simulink model "sch_2"  (R2022b)
settings: Solver=FixedStepAuto  StartTime=0.0  StopTime=3*t_final  FixedStep=1  RelTol=1e-3
values from neighbouring files (symbols this model uses):
  a = 7068e3    (= 7068000)    [prgBE_DSAS.m]
  Kp = lqr(Ap,Bp,eye(9),1e11*eye(3))    [prgBE_DSAS.m]
  n = sqrt(mu/a^3)    [prgBE_DSAS.m]
  X_init_chasseur = [x_init(2);y_init(2);z_init(2);Vx_init(2);Vy_init(2);Vz_init(2)]    [initialisation_a_distribuer.m]
  X_init_cible = [x_init(1);y_init(1);z_init(1);Vx_init(1);Vy_init(1);Vz_init(1)]    [initialisation_a_distribuer.m]
undefined symbols (not defined in the file or in its folder): ecc, inc, nu, W, w
settings Model: Creator=franc  LastModifiedBy=Utilisateur
settings DataIOCC: ReturnWorkspaceOutputs=off
settings OptimizationCC: ReuseModelBlockBuffer=on

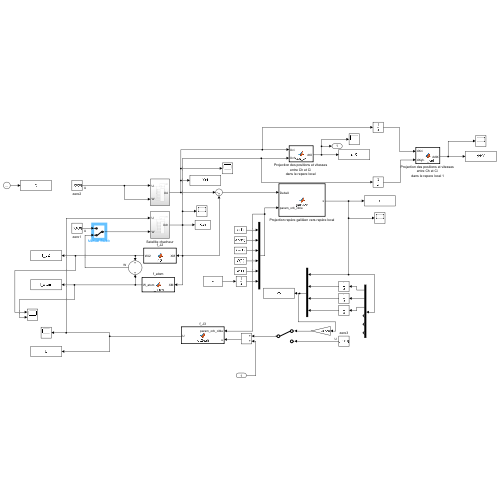
[thumbnail: Simulink's stored preview of the top-level diagram]
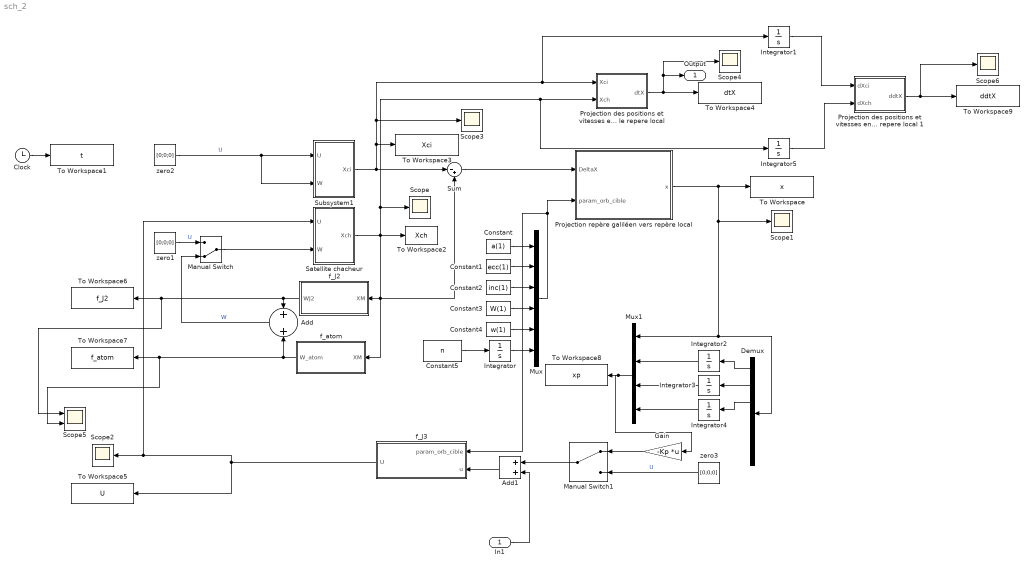
== system sch_2 ==
  In1 : Inport
  Add : Sum
  Add1 : Sum
  Clock : Clock
  Constant : Constant  Value=a(1)
  Constant1 : Constant  Value=ecc(1)
  Constant2 : Constant  Value=inc(1)
  Constant3 : Constant  Value=W(1)
  Constant4 : Constant  Value=w(1)
  Constant5 : Constant  Value=n
  Demux : Demux  Outputs=6
  Gain : Gain  Gain=-Kp  Multiplication=Matrix(K*u)
  Integrator : Integrator  InitialCondition=nu(1)
  Integrator{1..5} (5 alike) : Integrator
  Manual Switch : ManualSwitch  CurrentSetting=0
  Manual Switch1 : ManualSwitch
  Mux : Mux  Inputs=6
  Mux1 : Mux
  "Projection des positions et vitesses entre Ch et Ci dans le repere local " : MATLAB Function  TreatAsAtomicUnit=on
  Projection des positions et vitesses entre Ch et Ci dans le repere local 1 : MATLAB Function  TreatAsAtomicUnit=on
  Projection repère galiléen vers repère local : MATLAB Function  TreatAsAtomicUnit=on
  Satellite chacheur : Subsystem
  Scope{,1..4,6} (6 alike) : Scope
  Scope5 : Scope  NumInputPorts=2
  Subsystem1 : Subsystem
  Sum : Sum  Inputs=|-+
  To Workspace : ToWorkspace  VariableName=x  SampleTime=-1
  To Workspace1 : ToWorkspace  VariableName=t  SampleTime=-1
  To Workspace2 : ToWorkspace  VariableName=Xch  SampleTime=-1
  To Workspace3 : ToWorkspace  VariableName=Xci  SampleTime=-1
  To Workspace4 : ToWorkspace  VariableName=dtX  SampleTime=-1
  To Workspace5 : ToWorkspace  VariableName=U  SampleTime=-1
  To Workspace6 : ToWorkspace  VariableName=f_J2  SampleTime=-1
  To Workspace7 : ToWorkspace  VariableName=f_atom  SampleTime=-1
  To Workspace8 : ToWorkspace  VariableName=xp  SampleTime=-1
  To Workspace9 : ToWorkspace  VariableName=ddtX  SampleTime=-1
  f_J2 : MATLAB Function  TreatAsAtomicUnit=on
  f_J3 : MATLAB Function  TreatAsAtomicUnit=on
  f_atom : MATLAB Function  TreatAsAtomicUnit=on
  zero1 : Constant  Value=[0;0;0]
  zero2 : Constant  Value=[0;0;0]
  zero3 : Constant  Value=[0;0;0]
  Output : Outport
  wires:
  Integrator3/1 -> Mux1/3
  Integrator4/1 -> Mux1/4
  Gain/1 -> Manual Switch1/1
  Demux/3 -> Integrator4/1
  Projection repère galiléen vers repère local/1(x) -> Scope1/1, Demux/1, Mux1/1, To Workspace/1
  Demux/2 -> Integrator3/1
  Demux/1 -> Integrator2/1
  Constant1/1 -> Mux/2
  Constant/1 -> Mux/1
  zero1/1 -> Manual Switch/1  "U"
  zero2/1 -> Subsystem1/2(W), Subsystem1/1(U)  "U"
  Manual Switch/1 -> Satellite chacheur/2(W)
  Integrator/1 -> Mux/6
  Add/1 -> Manual Switch/2  "W"
  zero3/1 -> Manual Switch1/2  "U"
  "Projection des positions et vitesses entre Ch et Ci dans le repere local "/1(dtX) -> Output/1, Scope4/1, To Workspace4/1
  Mux1/1 -> Gain/1, To Workspace8/1
  Constant5/1 -> Integrator/1
  Constant3/1 -> Mux/4
  Clock/1 -> To Workspace1/1
  f_J3/1(U) -> Satellite chacheur/1(U), Scope2/1, To Workspace5/1
  Integrator2/1 -> Mux1/2
  Mux/1 -> f_J3/1(param_orb_cible), Projection repère galiléen vers repère local/2(param_orb_cible)
  f_J2/1(WJ2) -> Scope5/1, To Workspace6/1, Add/1
  Constant4/1 -> Mux/5
  f_atom/1(W_atom) -> Scope5/2, To Workspace7/1, Add/2
  Constant2/1 -> Mux/3
  Sum/1 -> Projection repère galiléen vers repère local/1(DeltaX)
  Integrator5/1 -> Projection des positions et vitesses entre Ch et Ci dans le repere local 1/2(dXch)
  Satellite chacheur/1(Xch) -> Integrator5/1, "Projection des positions et vitesses entre Ch et Ci dans le repere local "/2(Xch), Scope/1, f_atom/1(XM), Sum/2, f_J2/1(XM), To Workspace2/1
  Projection des positions et vitesses entre Ch et Ci dans le repere local 1/1(ddtX) -> Scope6/1, To Workspace9/1
  Subsystem1/1(Xci) -> Scope3/1, Integrator1/1, "Projection des positions et vitesses entre Ch et Ci dans le repere local "/1(Xci), To Workspace3/1, Sum/1
  Integrator1/1 -> Projection des positions et vitesses entre Ch et Ci dans le repere local 1/1(dXci)
  Add1/1 -> f_J3/2(u)
  In1/1 -> Add1/2
  Manual Switch1/1 -> Add1/1

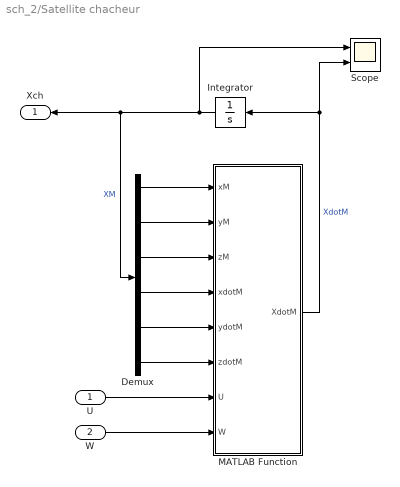
== system sch_2/Satellite chacheur ==
  U : Inport
  W : Inport  Port=2
  Demux : Demux  Outputs=6
  Integrator : Integrator  InitialCondition=X_init_chasseur
  MATLAB Function : MATLAB Function  TreatAsAtomicUnit=on
  Scope : Scope  NumInputPorts=2
  Xch : Outport
  wires:
  Demux/5 -> MATLAB Function/5(ydotM)
  Demux/1 -> MATLAB Function/1(xM)
  Demux/6 -> MATLAB Function/6(zdotM)
  MATLAB Function/1(XdotM) -> Scope/2, Integrator/1  "XdotM"
  Demux/4 -> MATLAB Function/4(xdotM)
  Integrator/1 -> Scope/1, Xch/1, Demux/1  "XM"
  Demux/2 -> MATLAB Function/2(yM)
  Demux/3 -> MATLAB Function/3(zM)
  U/1 -> MATLAB Function/7(U)
  W/1 -> MATLAB Function/8(W)

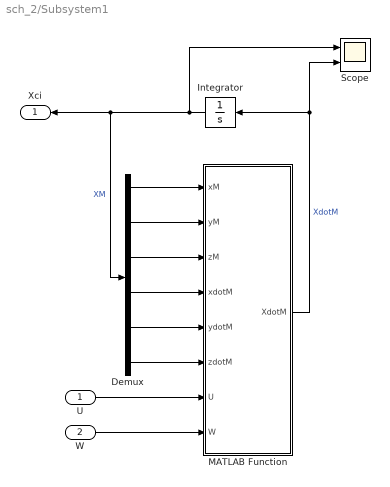
== system sch_2/Subsystem1 ==
  U : Inport
  W : Inport  Port=2
  Demux : Demux  Outputs=6
  Integrator : Integrator  InitialCondition=X_init_cible
  MATLAB Function : MATLAB Function  TreatAsAtomicUnit=on
  Scope : Scope  NumInputPorts=2
  Xci : Outport
  wires:
  Demux/5 -> MATLAB Function/5(ydotM)
  Demux/1 -> MATLAB Function/1(xM)
  Demux/6 -> MATLAB Function/6(zdotM)
  MATLAB Function/1(XdotM) -> Scope/2, Integrator/1  "XdotM"
  Demux/4 -> MATLAB Function/4(xdotM)
  Integrator/1 -> Scope/1, Xci/1, Demux/1  "XM"
  Demux/2 -> MATLAB Function/2(yM)
  Demux/3 -> MATLAB Function/3(zM)
  U/1 -> MATLAB Function/7(U)
  W/1 -> MATLAB Function/8(W)

== matlab function sch_2/Subsystem1/MATLAB Function ==
  data: xM input; yM input; zM input; xdotM input; ydotM input; zdotM input; XdotM output; U input; W input
function XdotM = f(xM,yM,zM,xdotM,ydotM,zdotM, U, W)
mu = 3.986e14; 
BW = [  zeros(3,3);
        eye(3)];

BU = [  eye(3);
        zeros(3,3)];


XdotM = [   xdotM;
            ydotM;
            zdotM;
            -mu/sqrt((xM^2 + yM^2 + zM^2)^3)*xM;
            -mu/sqrt((xM^2 + yM^2 + zM^2)^3)*yM;
            -mu/sqrt((xM^2 + yM^2 + zM^2)^3)*zM] + BU*U + BW*W;

== matlab function sch_2/Satellite chacheur/MATLAB Function ==
  data: xM input; yM input; zM input; xdotM input; ydotM input; zdotM input; XdotM output; U input; W input
function XdotM = f(xM,yM,zM,xdotM,ydotM,zdotM, U, W)
mu = 3.986e14; 
BW = [  zeros(3,3);
        eye(3)];

BU = [  zeros(3,3);  
        eye(3)     ];


XdotM = [   xdotM;
            ydotM;
            zdotM;
            -mu/sqrt((xM^2 + yM^2 + zM^2)^3)*xM;
            -mu/sqrt((xM^2 + yM^2 + zM^2)^3)*yM;
            -mu/sqrt((xM^2 + yM^2 + zM^2)^3)*zM] + BU*U + BW*W;

== matlab function sch_2/f_atom ==
  data: XM input; W_atom output
function W_atom = f_atom(XM)

rho_0 = 6.3e-13; 
rho = rho_0; 
S = 2; 
m = 191.1; 
CD = 2; 

W_atom = [  -rho*S*CD*sqrt(XM(4)^2+XM(5)^2+XM(6)^2)/2/m*XM(4)
            -rho*S*CD*sqrt(XM(4)^2+XM(5)^2+XM(6)^2)/2/m*XM(5)
            -rho*S*CD*sqrt(XM(4)^2+XM(5)^2+XM(6)^2)/2/m*XM(6) ];

== matlab function sch_2/f_J2 ==
  data: XM input; WJ2 output
function WJ2 = fJ2(XM)

mu = 3.986e14;          % constante gravitationnnelle 
J2 = 1.082616e-3;       % second harmonique 
Req = 6378e3;           % rayon terrestre (m)
WJ2 = 1/2*mu*J2*Req*Req*(3/sqrt(XM(1)^2+XM(2)^2+XM(3)^2)^4 - 15*XM(3)/sqrt(XM(1)^2+XM(2)^2+XM(3)^2)^6)*[XM(1);XM(2);XM(3)]/sqrt(XM(1)^2+XM(2)^2+XM(3)^2);

== matlab function sch_2/Projection repère galiléen vers repère local ==
  data: DeltaX input; x output; param_orb_cible input
function x = gali2loc(DeltaX,param_orb_cible)

mu = 3.986e14;

Delta_pos_gali = DeltaX(1:3);
Delta_vit_gali = DeltaX(4:6);
a1 = param_orb_cible(1);
ecc1 = param_orb_cible(2);
inc1 = param_orb_cible(3);
W1 = param_orb_cible(4);
w1 = param_orb_cible(5);
nu1 = param_orb_cible(6);

 P_gali2loc = [cos(W1)*cos(w1+nu1)-sin(W1)*cos(inc1)*sin(w1+nu1),...
     cos(W1)*sin(w1+nu1)+sin(W1)*cos(inc1)*cos(w1+nu1),...
     sin(W1)*sin(inc1);...
     -sin(W1)*cos(w1+nu1)-cos(W1)*cos(inc1)*sin(w1+nu1),...
     -sin(W1)*sin(w1+nu1)+cos(W1)*cos(inc1)*cos(w1+nu1),...
     cos(W1)*sin(inc1);...
     sin(inc1)*sin(w1+nu1),...
     -sin(inc1)*cos(w1+nu1),...
     cos(inc1)];
 Delta_pos_loc=(P_gali2loc)*Delta_pos_gali;
 Delta_vit_loc=(P_gali2loc)*Delta_vit_gali;

 Omega_R1_R0=[0;0;sqrt(mu/(a1^3))];
 Delta_vit_loc_R1=Delta_vit_loc+cross(Delta_pos_loc,Omega_R1_R0);
 
x=[Delta_pos_loc;Delta_vit_loc_R1];

== matlab function sch_2/f_J3 ==
  data: param_orb_cible input; u input; U output
function U = loc2gali(param_orb_cible,u)

mu = 3.986e14;

ux_loc = u(1);
uy_loc = u(2);
uz_loc = u(3);
a1 = param_orb_cible(1);
ecc1 = param_orb_cible(2);
inc1 = param_orb_cible(3);
W1 = param_orb_cible(4);
w1 = param_orb_cible(5);
nu1 = param_orb_cible(6);

 uloc=[ux_loc;uy_loc;uz_loc];
 P_gali2loc = [cos(W1)*cos(w1+nu1)-sin(W1)*cos(inc1)*sin(w1+nu1),...
     cos(W1)*sin(w1+nu1)+sin(W1)*cos(inc1)*cos(w1+nu1),...
     sin(W1)*sin(inc1);...
     -sin(W1)*cos(w1+nu1)-cos(W1)*cos(inc1)*sin(w1+nu1),...
     -sin(W1)*sin(w1+nu1)+cos(W1)*cos(inc1)*cos(w1+nu1),...
     cos(W1)*sin(inc1);...
     sin(inc1)*sin(w1+nu1),...
     -sin(inc1)*cos(w1+nu1),...
     cos(inc1)];
 ugali=(P_gali2loc')*uloc;

U=ugali;

== matlab function sch_2/Projection des positions et vitesses entre Ch et Ci dans le repere local  ==
  data: Xci input; Xch input; dtX output
function dtX = pos_vel(Xci,Xch)

dtX = Xch-Xci;

== matlab function sch_2/Projection des positions et vitesses entre Ch et Ci dans le repere local 1 ==
  data: dXci input; dXch input; ddtX output
function ddtX = pos_vel(dXci,dXch)

ddtX = dXch-dXci;
